simulink library "UAV_Control"  (R2018a)
settings: Solver=ode45  StartTime=0.0  StopTime=10.0  RelTol=1e-3  EnableMultiTasking=on
undefined symbols (not defined in the file or in its folder): alpha, dc_M_z, delta, Epsilon, g, Gamma, gamma_0, gamma_d_z, h, k, K, Ky, L, magnitude, mu1, mu2, nu, omega0, omega1, omega2, Phi0, Psi0, Rate, Rho_L, Rho_M, RPM_per, Sat, t0, t1, Tau, theta, theta0, Theta0, theta_0, theta_dot_M, theta_Max, theta_Min, Thrust_per, Tm, v, V0, X0, Xmax, Xmin, zeta1, zeta2, Zg
libraries: simulink x12, $bdroot x7
(part 2 of 2)

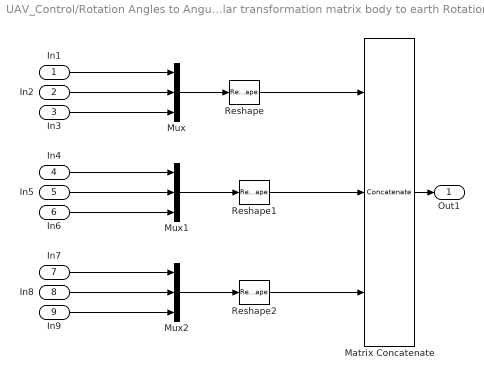
== system UAV_Control/Rotation Angles to Angular transformation matrix body to earth Rotation Order: ZXY/Subsystem ==
  In1 : Inport
  In2 : Inport  Port=2
  In3 : Inport  Port=3
  In4 : Inport  Port=4
  In5 : Inport  Port=5
  In6 : Inport  Port=6
  In7 : Inport  Port=7
  In8 : Inport  Port=8
  In9 : Inport  Port=9
  Matrix Concatenate : Concatenate  NumInputs=3  Mode=Multidimensional array  ConcatenateDimension=2
  Mux : Mux  Inputs=3
  Mux1 : Mux  Inputs=3
  Mux2 : Mux  Inputs=3
  Reshape : Reshape  OutputDimensionality=Column vector (2-D)
  Reshape1 : Reshape  OutputDimensionality=Column vector (2-D)
  Reshape2 : Reshape  OutputDimensionality=Column vector (2-D)
  Out1 : Outport
  wires:
  Reshape1/1 -> Matrix Concatenate/2
  Mux1/1 -> Reshape1/1
  Reshape/1 -> Matrix Concatenate/1
  Reshape2/1 -> Matrix Concatenate/3
  Matrix Concatenate/1 -> Out1/1
  Mux2/1 -> Reshape2/1
  Mux/1 -> Reshape/1
  In1/1 -> Mux/1
  In2/1 -> Mux/2
  In3/1 -> Mux/3
  In4/1 -> Mux1/1
  In5/1 -> Mux1/2
  In6/1 -> Mux1/3
  In7/1 -> Mux2/1
  In8/1 -> Mux2/2
  In9/1 -> Mux2/3

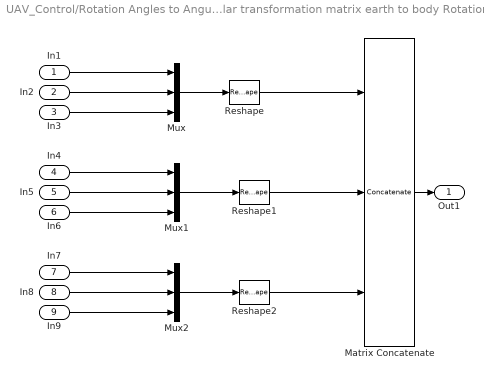
== system UAV_Control/Rotation Angles to Angular transformation matrix earth to body Rotation Order: ZXY/Subsystem ==
  In1 : Inport
  In2 : Inport  Port=2
  In3 : Inport  Port=3
  In4 : Inport  Port=4
  In5 : Inport  Port=5
  In6 : Inport  Port=6
  In7 : Inport  Port=7
  In8 : Inport  Port=8
  In9 : Inport  Port=9
  Matrix Concatenate : Concatenate  NumInputs=3  Mode=Multidimensional array  ConcatenateDimension=2
  Mux : Mux  Inputs=3
  Mux1 : Mux  Inputs=3
  Mux2 : Mux  Inputs=3
  Reshape : Reshape  OutputDimensionality=Column vector (2-D)
  Reshape1 : Reshape  OutputDimensionality=Column vector (2-D)
  Reshape2 : Reshape  OutputDimensionality=Column vector (2-D)
  Out1 : Outport
  wires:
  In9/1 -> Mux2/3
  In8/1 -> Mux2/2
  In7/1 -> Mux2/1
  In6/1 -> Mux1/3
  In5/1 -> Mux1/2
  In4/1 -> Mux1/1
  In3/1 -> Mux/3
  In2/1 -> Mux/2
  In1/1 -> Mux/1
  Mux/1 -> Reshape/1
  Mux2/1 -> Reshape2/1
  Matrix Concatenate/1 -> Out1/1
  Reshape2/1 -> Matrix Concatenate/3
  Reshape/1 -> Matrix Concatenate/1
  Mux1/1 -> Reshape1/1
  Reshape1/1 -> Matrix Concatenate/2

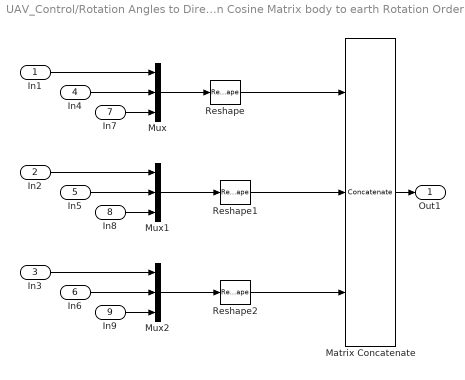
== system UAV_Control/Rotation Angles to Direction Cosine Matrix body to earth Rotation Order: ZXY/Subsystem ==
  In1 : Inport
  In2 : Inport  Port=2
  In3 : Inport  Port=3
  In4 : Inport  Port=4
  In5 : Inport  Port=5
  In6 : Inport  Port=6
  In7 : Inport  Port=7
  In8 : Inport  Port=8
  In9 : Inport  Port=9
  Matrix Concatenate : Concatenate  NumInputs=3  Mode=Multidimensional array  ConcatenateDimension=2
  Mux : Mux  Inputs=3
  Mux1 : Mux  Inputs=3
  Mux2 : Mux  Inputs=3
  Reshape : Reshape  OutputDimensionality=Column vector (2-D)
  Reshape1 : Reshape  OutputDimensionality=Column vector (2-D)
  Reshape2 : Reshape  OutputDimensionality=Column vector (2-D)
  Out1 : Outport
  wires:
  In9/1 -> Mux2/3
  In6/1 -> Mux2/2
  In3/1 -> Mux2/1
  In5/1 -> Mux1/2
  In8/1 -> Mux1/3
  In2/1 -> Mux1/1
  In7/1 -> Mux/3
  In4/1 -> Mux/2
  Mux/1 -> Reshape/1
  In1/1 -> Mux/1
  Mux2/1 -> Reshape2/1
  Matrix Concatenate/1 -> Out1/1
  Reshape2/1 -> Matrix Concatenate/3
  Reshape/1 -> Matrix Concatenate/1
  Mux1/1 -> Reshape1/1
  Reshape1/1 -> Matrix Concatenate/2

== system UAV_Control/sensor/delay ==
  u : Inport
  Memory{1..4,10} (5 alike) : Memory
  y : Outport
  wires:
  Memory4/1 -> Memory10/1
  Memory2/1 -> Memory3/1
  Memory1/1 -> Memory2/1
  Memory10/1 -> Memory1/1
  u/1 -> Memory4/1
  Memory3/1 -> y/1

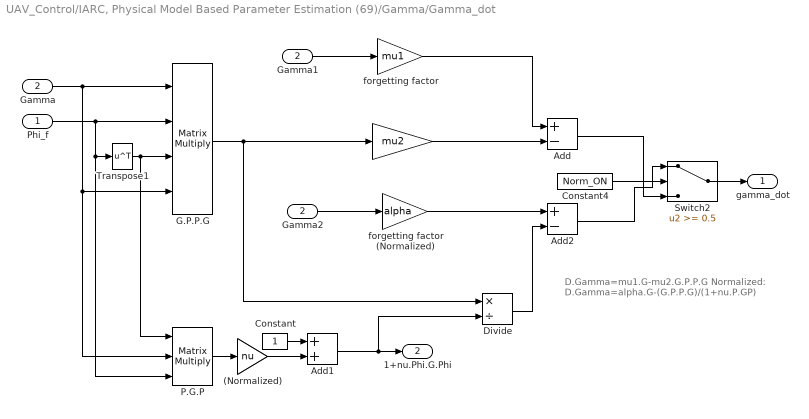
== system UAV_Control/IARC, Physical Model Based Parameter Estimation (69)/Gamma/Gamma_dot ==
  note: D.Gamma=mu1.G-mu2.G.P.P.G
      |
      | Normalized:
      | D.Gamma=alpha.G-(G.P.P.G)/(1+nu.P.GP)
  Phi_f : Inport
  Gamma : Inport  Port=2
  " " : Gain  Gain=mu2
  "  (Normalized)" : Gain  Gain=nu
  Add : Sum  Inputs=+-
  Add1 : Sum
  Add2 : Sum  Inputs=+-
  Constant : Constant
  Constant4 : Constant  Value=Norm_ON
  Divide : Product  Inputs=*/
  G.P.P.G : Product  Inputs=4  Multiplication=Matrix(*)
  Gamma1 : InportShadow  Port=2
  Gamma2 : InportShadow  Port=2
  P.G.P : Product  Inputs=3  Multiplication=Matrix(*)
  Switch2 : Switch  Threshold=0.5
  Transpose1 : Math  Operator=transpose  SaturateOnIntegerOverflow=on
  "forgetting factor " : Gain  Gain=mu1
  forgetting factor (Normalized) : Gain  Gain=alpha
  gamma_dot : Outport
  " 1+nu.Phi.G.Phi" : Outport  Port=2
  wires:
  Gamma1/1 -> "forgetting factor "/1
  " "/1 -> Add/2
  forgetting factor (Normalized)/1 -> Add2/1
  Divide/1 -> Add2/2
  Switch2/1 -> gamma_dot/1
  Add/1 -> Switch2/3
  Constant4/1 -> Switch2/2
  Add2/1 -> Switch2/1
  Gamma2/1 -> forgetting factor (Normalized)/1
  Add1/1 -> " 1+nu.Phi.G.Phi"/1, Divide/2
  P.G.P/1 -> "  (Normalized)"/1
  Constant/1 -> Add1/1
  G.P.P.G/1 -> Divide/1, " "/1
  "forgetting factor "/1 -> Add/1
  Gamma/1 -> G.P.P.G/4, P.G.P/2, G.P.P.G/1
  Transpose1/1 -> G.P.P.G/3, P.G.P/1
  Phi_f/1 -> G.P.P.G/2, Transpose1/1, P.G.P/3
  "  (Normalized)"/1 -> Add1/2

== system UAV_Control/IARC, Physical Model Based Parameter Estimation (69)/Gamma/vDv ==
  In1 : Inport
  Product2 : Product  Inputs=3  Multiplication=Matrix(*)
  Transpose2 : Math  Operator=transpose  SaturateOnIntegerOverflow=on
  eigenvector of Gamm_max : Constant  Value=v
  Out1 : Outport
  wires:
  Product2/1 -> Out1/1
  eigenvector of Gamm_max/1 -> Product2/3, Transpose2/1
  In1/1 -> Product2/2
  Transpose2/1 -> Product2/1
